simulink model "nonlinear_system"  (R2024b)
settings: Solver=VariableStepAuto  StartTime=0.0  StopTime=Tfin  MaxStep=0.2  RelTol=1e-3
values from neighbouring files (symbols this model uses):
  a = pi*r^2    (= 78.5398163397)    [script_project.m]
  Cd = 1.2    [script_project.m]
  g = 9.81    [script_project.m]
  h = 70    [script_project.m]
  J = (1/12)*m*(b^2 + h^2)    (= 208333333.333)    [script_project.m]
  m = 500000    [script_project.m]
  rho = 1.225    [script_project.m]
  u0 = [u1eq u2eq u3eq]'    [script_project.m]
  z0 = [x2eq x2doteq thetaeq thetadoteq]'    [script_project.m]
settings Model: Creator=martinhaugen  LastModifiedBy=martinhaugen
settings DataIOCC: ExternalInput=[t, u0]

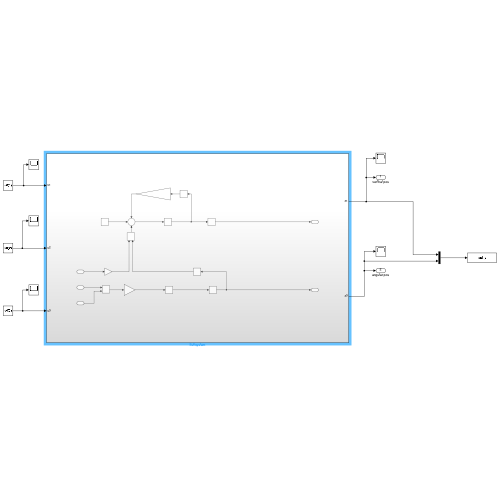
[thumbnail: Simulink's stored preview of the top-level diagram]
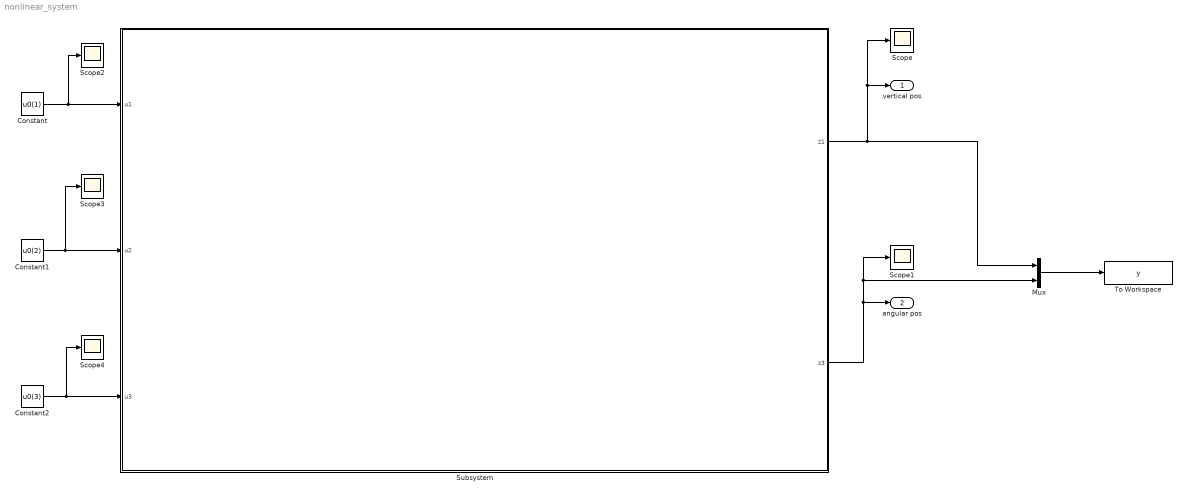
== system nonlinear_system ==
  Constant : Constant  Value=u0(1)  SampleTime=-1
  Constant1 : Constant  Value=u0(2)  SampleTime=-1
  Constant2 : Constant  Value=u0(3)  SampleTime=-1
  Mux : Mux  Inputs=2
  Scope{,1..4} (5 alike) : Scope
  Subsystem : Subsystem
  To Workspace : ToWorkspace  VariableName=y  SaveFormat=Timeseries  SampleTime=-1
  vertical pos : Outport
  angular pos : Outport  Port=2
  wires:
  Constant/1 -> Scope2/1, Subsystem/1(u1)
  Constant1/1 -> Scope3/1, Subsystem/2(u2)
  Constant2/1 -> Scope4/1, Subsystem/3(u3)
  Subsystem/1(z1) -> Scope/1, vertical pos/1, Mux/1
  Mux/1 -> To Workspace/1
  Subsystem/2(z3) -> Scope1/1, Mux/2, angular pos/1

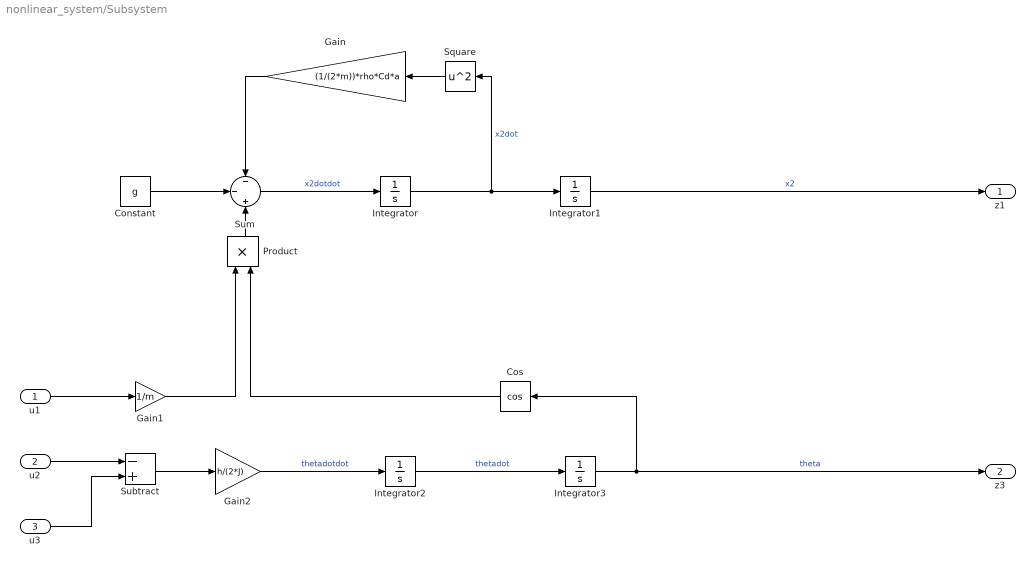
== system nonlinear_system/Subsystem ==
  u1 : Inport
  u2 : Inport  Port=2
  u3 : Inport  Port=3
  Constant : Constant  Value=g
  Cos : Trigonometry  Operator=cos
  Gain : Gain  Gain=(1/(2*m))*rho*Cd*a
  Gain1 : Gain  Gain=1/m
  Gain2 : Gain  Gain=h/(2*J)
  Integrator : Integrator  InitialCondition=z0(2)
  Integrator1 : Integrator  InitialCondition=z0(1)
  Integrator2 : Integrator  InitialCondition=z0(4)
  Integrator3 : Integrator  InitialCondition=z0(3)
  Product : Product
  Square : Math  Operator=square
  Subtract : Sum  Inputs=-+
  Sum : Sum  Inputs=-|-|+
  z1 : Outport
  z3 : Outport  Port=2
  wires:
  u2/1 -> Subtract/1
  Constant/1 -> Sum/2
  Square/1 -> Gain/1
  Product/1 -> Sum/3
  Subtract/1 -> Gain2/1
  Integrator/1 -> Integrator1/1, Square/1  "x2dot"
  Gain2/1 -> Integrator2/1  "thetadotdot"
  Cos/1 -> Product/2
  u3/1 -> Subtract/2
  Integrator2/1 -> Integrator3/1  "thetadot"
  u1/1 -> Gain1/1
  Gain/1 -> Sum/1
  Sum/1 -> Integrator/1  "x2dotdot"
  Gain1/1 -> Product/1
  Integrator3/1 -> z3/1, Cos/1  "theta"
  Integrator1/1 -> z1/1  "x2"
